simulink subsystem "motores"  (R2023b)
settings: Solver=VariableStepAuto  StartTime=0.0  StopTime=10.0  RelTol=1e-3
libraries: arduinolib x6, simulink x4
settings Model: Creator=Usuario_UMA  LastModifiedBy=Carlos

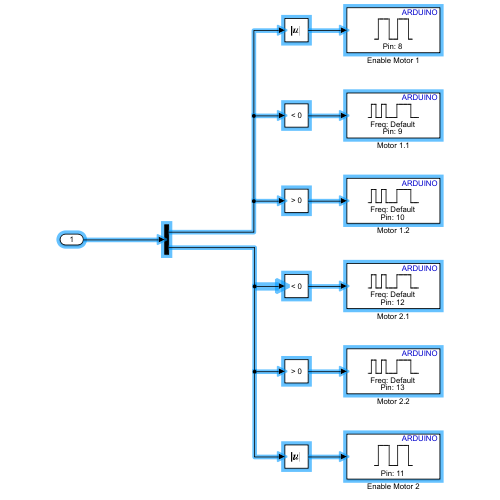
[thumbnail: Simulink's stored preview of the top-level diagram]
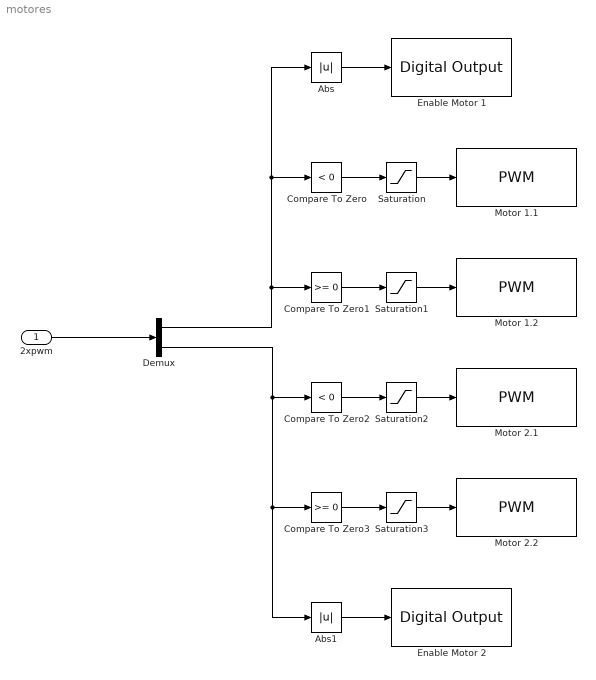
== system motores ==
  2xpwm : Inport  OutDataTypeStr=uint8
  Abs : Abs  SaturateOnIntegerOverflow=off
  Abs1 : Abs  SaturateOnIntegerOverflow=off
  Compare To Zero : simulink/Logic and Bit Operations/Compare To Zero  relop=<  OutDataTypeStr=uint8
  Compare To Zero1 : simulink/Logic and Bit Operations/Compare To Zero  relop=>=  OutDataTypeStr=uint8
  Compare To Zero2 : simulink/Logic and Bit Operations/Compare To Zero  relop=<  OutDataTypeStr=uint8
  Compare To Zero3 : simulink/Logic and Bit Operations/Compare To Zero  relop=>=  OutDataTypeStr=uint8
  Demux : Demux  Outputs=2
  Enable Motor 1 : arduinolib/Digital Output  pinNumber=8  Direction=output  blockPlatform=arduino
  Enable Motor 2 : arduinolib/Digital Output  pinNumber=11  Direction=output  blockPlatform=arduino
  Motor 1.1 : arduinolib/PWM  pinNumber=9  frequencyType=Default  desiredFrequency=490.2  achievableFrequency=490.2
  Motor 1.2 : arduinolib/PWM  pinNumber=10  frequencyType=Default  desiredFrequency=490.2  achievableFrequency=490.2
  Motor 2.1 : arduinolib/PWM  pinNumber=12  frequencyType=Default  desiredFrequency=490.2  achievableFrequency=490.2
  Motor 2.2 : arduinolib/PWM  pinNumber=13  frequencyType=Default  desiredFrequency=490.2  achievableFrequency=490.2
  Saturation : Saturate  UpperLimit=0  LowerLimit=-255
  Saturation1 : Saturate  UpperLimit=255  LowerLimit=0
  Saturation2 : Saturate  UpperLimit=0  LowerLimit=-255
  Saturation3 : Saturate  UpperLimit=255  LowerLimit=0
  wires:
  Compare To Zero3/1 -> Saturation3/1
  Abs1/1 -> Enable Motor 2/1
  Compare To Zero1/1 -> Saturation1/1
  Compare To Zero2/1 -> Saturation2/1
  Compare To Zero/1 -> Saturation/1
  2xpwm/1 -> Demux/1
  Demux/1 -> Abs/1, Compare To Zero/1, Compare To Zero1/1
  Abs/1 -> Enable Motor 1/1
  Demux/2 -> Compare To Zero2/1, Compare To Zero3/1, Abs1/1
  Saturation/1 -> Motor 1.1/1
  Saturation1/1 -> Motor 1.2/1
  Saturation2/1 -> Motor 2.1/1
  Saturation3/1 -> Motor 2.2/1
